simulink model "bloques_realestados"  (R2021a)
settings: Solver=ode4  StartTime=0.0  StopTime=5  FixedStep=1e-4  RelTol=1e-3
values from neighbouring files (symbols this model uses):
  A = [ ... (first row only)    [disenio_realimentacion_estado.m]
  B = [ B_sb; 0; 0; 0 ]    [disenio_realimentacion_estado.m]
  C = [ ... (first row only)    [disenio_realimentacion_estado.m]
  Kc = place(A, B, polos_c)    [disenio_realimentacion_estado.m]
undefined symbols (not defined in the file or in its folder): Fc, Lc
libraries: simulink x1
settings Model: Creator=rocio  LastModifiedBy=rocio

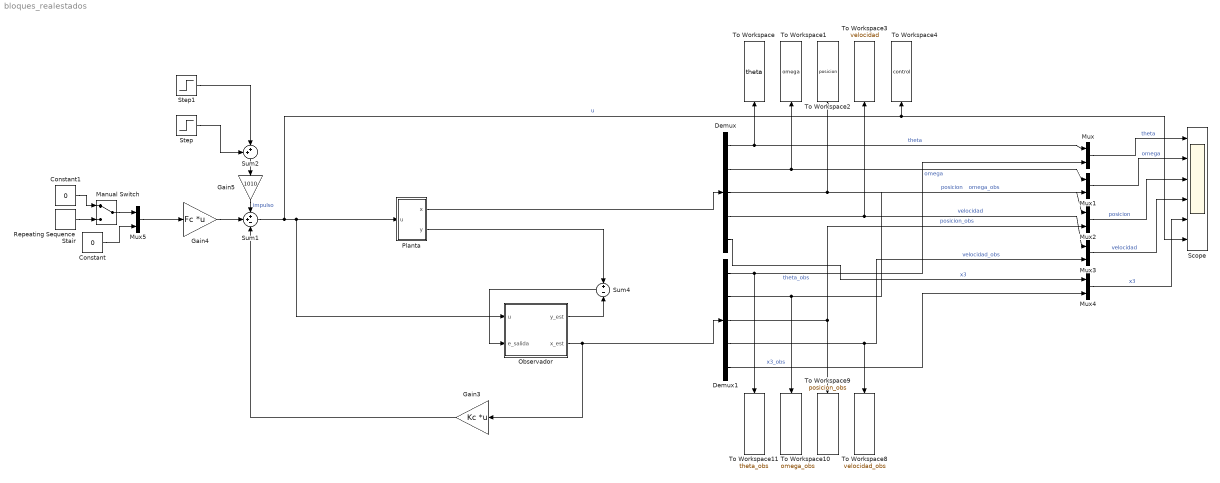
== system bloques_realestados ==
  Constant : Constant  Value=0
  Constant1 : Constant  Value=0
  Demux : Demux  Outputs=5
  Demux1 : Demux  Outputs=5
  Gain3 : Gain  Gain=Kc  Multiplication=Matrix(K*u) (u vector)
  Gain4 : Gain  Gain=Fc  Multiplication=Matrix(K*u) (u vector)
  Gain5 : Gain  Gain=1010
  Manual Switch : ManualSwitch
  Mux{,1..5} (6 alike) : Mux  Inputs=2
  Observador : Subsystem
  Planta : Subsystem
  Repeating Sequence Stair : simulink/Sources/Repeating Sequence Stair  OutValues=[8 -6 0]  tsamp=5.98  OutMin=[]  OutMax=[]  OutDataTypeStr=double  OutputDataTypeScalingMode=double  OutDataType=fixdt(0,8)  ConRadixGroup=Best Precision: Vector-wise  OutScaling=2^-12
  Scope : Scope  NumInputPorts=6
  Step : Step  Time=0.85  After=-1  SampleTime=0
  Step1 : Step  Time=0  SampleTime=0
  Sum1 : Sum  Inputs=++-
  Sum2 : Sum  Inputs=++|
  Sum4 : Sum  Inputs=+|-
  To Workspace : ToWorkspace  VariableName=theta  SampleTime=-1
      settings: Save2DSignal=2-D array (concatenate along first dimension)
  To Workspace1 : ToWorkspace  VariableName=omega  SampleTime=-1
      settings: Save2DSignal=2-D array (concatenate along first dimension)
  To Workspace10 : ToWorkspace  VariableName=omega_obs  SampleTime=-1
      settings: Save2DSignal=2-D array (concatenate along first dimension)
  To Workspace11 : ToWorkspace  VariableName=theta_obs  SampleTime=-1
      settings: Save2DSignal=2-D array (concatenate along first dimension)
  To Workspace2 : ToWorkspace  VariableName=posicion  SampleTime=-1
      settings: Save2DSignal=2-D array (concatenate along first dimension)
  To Workspace3 : ToWorkspace  VariableName=velocidad  SampleTime=-1
      settings: Save2DSignal=2-D array (concatenate along first dimension)
  To Workspace4 : ToWorkspace  VariableName=control  SampleTime=-1
      settings: Save2DSignal=2-D array (concatenate along first dimension)
  To Workspace8 : ToWorkspace  VariableName=velocidad_obs  SampleTime=-1
      settings: Save2DSignal=2-D array (concatenate along first dimension)
  To Workspace9 : ToWorkspace  VariableName=posicion_obs  SampleTime=-1
      settings: Save2DSignal=2-D array (concatenate along first dimension)
  wires:
  Sum1/1 -> To Workspace4/1, Scope/6, Observador/1(u), Planta/1(u)  "u"
  Mux5/1 -> Gain4/1
  Gain4/1 -> Sum1/2
  Gain3/1 -> Sum1/3
  Step1/1 -> Sum2/2
  Step/1 -> Sum2/1
  Sum2/1 -> Gain5/1
  Gain5/1 -> Sum1/1  "impulso"
  Demux/1 -> Mux/1, To Workspace/1  "theta"
  Demux1/1 -> To Workspace11/1, Mux/2  "theta_obs"
  Demux/2 -> Mux1/1, To Workspace1/1  "omega"
  Demux1/2 -> To Workspace10/1, Mux1/2  "omega_obs"
  Demux/3 -> To Workspace2/1, Mux2/1  "posicion"
  Demux1/3 -> Mux2/2, To Workspace9/1  "posicion_obs"
  Demux/4 -> To Workspace3/1, Mux3/1  "velocidad"
  Demux1/4 -> To Workspace8/1, Mux3/2  "velocidad_obs"
  Mux/1 -> Scope/1  "theta"
  Mux1/1 -> Scope/2  "omega"
  Mux2/1 -> Scope/3  "posicion"
  Mux3/1 -> Scope/4  "velocidad"
  Mux4/1 -> Scope/5  "x3"
  Demux/5 -> Mux4/1  "x3"
  Demux1/5 -> Mux4/2  "x3_obs"
  Observador/2(x_est) -> Gain3/1, Demux1/1
  Sum4/1 -> Observador/2(e_salida)
  Observador/1(y_est) -> Sum4/2
  Planta/1(x) -> Demux/1
  Planta/2(y) -> Sum4/1
  Constant/1 -> Mux5/2
  Constant1/1 -> Manual Switch/1
  Repeating Sequence Stair/1 -> Manual Switch/2
  Manual Switch/1 -> Mux5/1

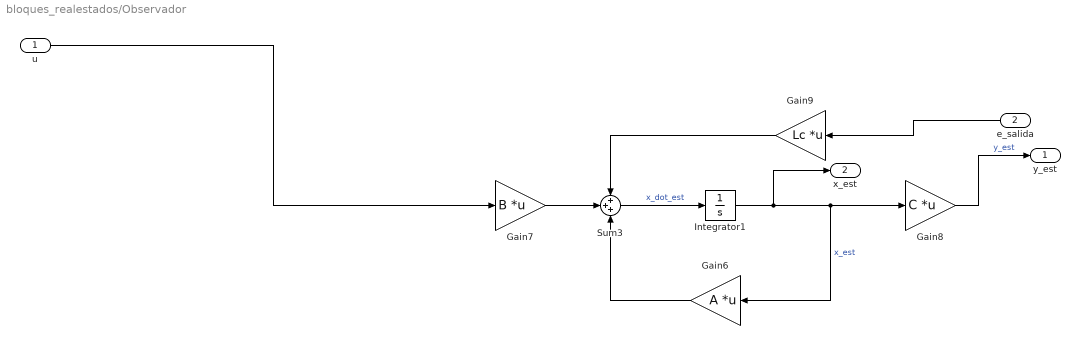
== system bloques_realestados/Observador ==
  u : Inport
  e_salida : Inport  Port=2
  Gain6 : Gain  Gain=A  Multiplication=Matrix(K*u) (u vector)
  Gain7 : Gain  Gain=B  Multiplication=Matrix(K*u) (u vector)
  Gain8 : Gain  Gain=C  Multiplication=Matrix(K*u) (u vector)
  Gain9 : Gain  Gain=Lc  Multiplication=Matrix(K*u) (u vector)
  Integrator1 : Integrator
  Sum3 : Sum  Inputs=+++
  y_est : Outport
  x_est : Outport  Port=2
  wires:
  Gain9/1 -> Sum3/1
  u/1 -> Gain7/1
  Sum3/1 -> Integrator1/1  "x_dot_est"
  e_salida/1 -> Gain9/1
  Gain6/1 -> Sum3/3
  Gain8/1 -> y_est/1  "y_est"
  Gain7/1 -> Sum3/2
  Integrator1/1 -> Gain6/1, Gain8/1, x_est/1  "x_est"

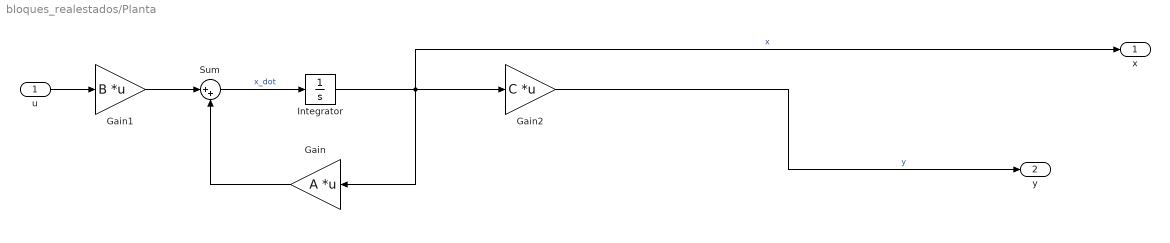
== system bloques_realestados/Planta ==
  u : Inport
  Gain : Gain  Gain=A  Multiplication=Matrix(K*u) (u vector)
  Gain1 : Gain  Gain=B  Multiplication=Matrix(K*u) (u vector)
  Gain2 : Gain  Gain=C  Multiplication=Matrix(K*u) (u vector)
  Integrator : Integrator
  Sum : Sum  Inputs=|++
  x : Outport
  y : Outport  Port=2
  wires:
  Gain1/1 -> Sum/1
  u/1 -> Gain1/1
  Gain/1 -> Sum/2
  Integrator/1 -> x/1, Gain2/1, Gain/1  "x"
  Sum/1 -> Integrator/1  "x_dot"
  Gain2/1 -> y/1  "y"
